simulink model "My_Nonlinear_Quaternions"  (R2021b)
settings: Solver=VariableStepAuto  StartTime=0.0  StopTime=simTime  RelTol=1e-3
undefined symbols (not defined in the file): b, D, g, k, L, m, MoI, omega, p, p_dot, quat, RPM, TakeStep
settings Model: Creator=Wojciech  LastModifiedBy=tanzc

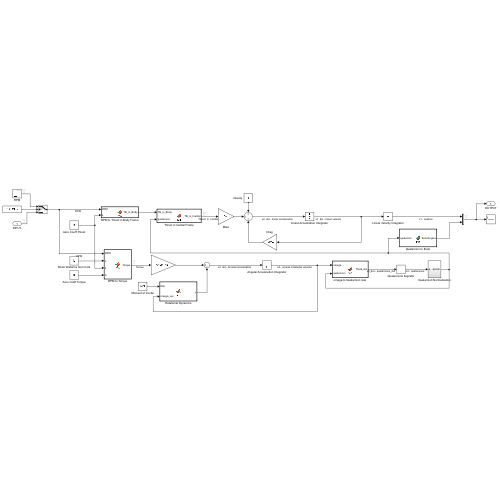
[thumbnail: Simulink's stored preview of the top-level diagram]
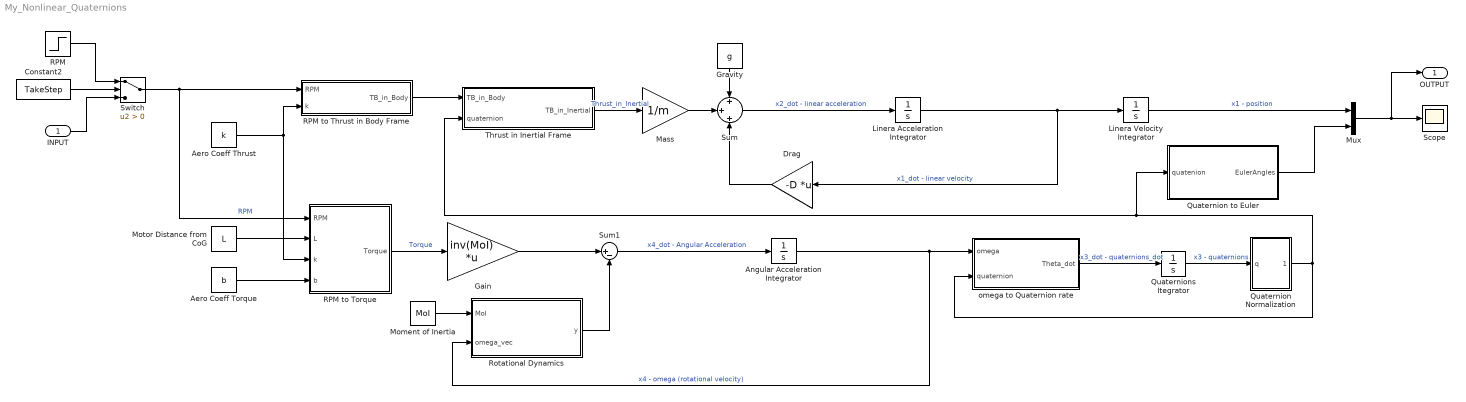
== system My_Nonlinear_Quaternions ==
  INPUT : Inport  PortDimensions=4
  Aero Coeff Thrust : Constant  Value=k
  Aero Coeff Torque : Constant  Value=b
  Angular Acceleration Integrator : Integrator  Priority=4  InitialCondition=omega
  Constant2 : Constant  Value=TakeStep
  Drag : Gain  Gain=-D  Multiplication=Matrix(K*u)
  Gain : Gain  Gain=inv(MoI)  Multiplication=Matrix(K*u)
  Gravity : Constant  Value=g  VectorParams1D=off
  Linera Acceleration Integrator : Integrator  Priority=2  InitialCondition=p_dot
  Linera Velocity Integrator : Integrator  Priority=1  InitialCondition=p
  Mass : Gain  Gain=1/m
  Moment of Inertia : Constant  Value=MoI  VectorParams1D=off
  Motor Distance from CoG : Constant  Value=L
  Mux : Mux  Inputs=2
  Quaternion Normalization : Subsystem
  Quaternion to Euler : MATLAB Function  TreatAsAtomicUnit=on
  Quaternions Itegrator : Integrator  Priority=3  InitialCondition=quat
  RPM : Step  Time=0  After=RPM  SampleTime=0
  RPM to Thrust in Body Frame : MATLAB Function  TreatAsAtomicUnit=on
  RPM to Torque : MATLAB Function  TreatAsAtomicUnit=on
  Rotational Dynamics : MATLAB Function  TreatAsAtomicUnit=on
  Scope : Scope
  Sum : Sum  Inputs=+|+|+
  Sum1 : Sum  Inputs=|+-
  Switch : Switch  Criteria=u2 > Threshold
  Thrust in Inertial Frame : MATLAB Function  TreatAsAtomicUnit=on
  "omega to Quaternion rate " : MATLAB Function  TreatAsAtomicUnit=on
  OUTPUT : Outport
  wires:
  Linera Velocity Integrator/1 -> Mux/1  "x1 - position"
  Linera Acceleration Integrator/1 -> Drag/1, Linera Velocity Integrator/1  "x1_dot - linear velocity"
  Sum/1 -> Linera Acceleration Integrator/1  "x2_dot - linear acceleration"
  Gravity/1 -> Sum/1
  RPM to Thrust in Body Frame/1(TB_in_Body) -> Thrust in Inertial Frame/1(TB_in_Body)
  Aero Coeff Thrust/1 -> RPM to Thrust in Body Frame/2(k), RPM to Torque/3(k)
  Thrust in Inertial Frame/1(TB_in_Inertial) -> Mass/1  "Thrust_in_Inertial"
  Mass/1 -> Sum/2
  Drag/1 -> Sum/3
  Motor Distance from CoG/1 -> RPM to Torque/2(L)
  Aero Coeff Torque/1 -> RPM to Torque/4(b)
  RPM to Torque/1(Torque) -> Gain/1  "Torque"
  Gain/1 -> Sum1/1
  Rotational Dynamics/1(y) -> Sum1/2
  Moment of Inertia/1 -> Rotational Dynamics/1(MoI)
  Sum1/1 -> Angular Acceleration Integrator/1  "x4_dot - Angular Acceleration"
  Angular Acceleration Integrator/1 -> "omega to Quaternion rate "/1(omega), Rotational Dynamics/2(omega_vec)  "x4 - omega (rotational velocity)"
  "omega to Quaternion rate "/1(Theta_dot) -> Quaternions Itegrator/1  "x3_dot - quaternions_dot"
  Quaternions Itegrator/1 -> Quaternion Normalization/1(q)  "x3 - quaternions"
  Mux/1 -> OUTPUT/1, Scope/1
  Constant2/1 -> Switch/2
  INPUT/1 -> Switch/3
  RPM/1 -> Switch/1
  Switch/1 -> RPM to Thrust in Body Frame/1(RPM), RPM to Torque/1(RPM)  "RPM"
  Quaternion Normalization/1(qnorm) -> Quaternion to Euler/1(quatenion), Thrust in Inertial Frame/2(quaternion), "omega to Quaternion rate "/2(quaternion)
  Quaternion to Euler/1(EulerAngles) -> Mux/2

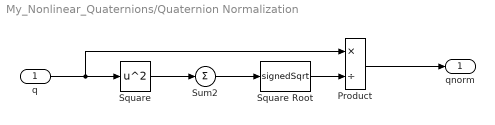
== system My_Nonlinear_Quaternions/Quaternion Normalization ==
  q : Inport  PortDimensions=4
  Product : Product  Inputs=*/
  Square : Math  Operator=square  SaturateOnIntegerOverflow=on
  Square Root : Sqrt  Operator=signedSqrt  SaturateOnIntegerOverflow=on
  Sum2 : Sum  Inputs=1
  qnorm : Outport  PortDimensions=4
  wires:
  Square Root/1 -> Product/2
  q/1 -> Product/1, Square/1
  Square/1 -> Sum2/1
  Sum2/1 -> Square Root/1
  Product/1 -> qnorm/1

== matlab function My_Nonlinear_Quaternions/RPM to Thrust in Body Frame ==
  data: RPM input; TB_in_Body output; k input
function TB_in_Body = fcn(RPM, k)
TB_in_Body = k * [0; 0; RPM'*RPM];

== matlab function My_Nonlinear_Quaternions/Thrust in Inertial Frame ==
  data: TB_in_Body input; quaternion input; TB_in_Inertial output
function TB_in_Inertial = fcn(TB_in_Body, quaternion)

% quaternion = [q0, q1, q2, q3]

q0 = quaternion(1);
q1 = quaternion(2);
q2 = quaternion(3);
q3 = quaternion(4);

R = quat2rotm([q0, q1, q2, q3]);

TB_in_Inertial = R*TB_in_Body;

== matlab function My_Nonlinear_Quaternions/RPM to Torque ==
  data: RPM input; Torque output; L input; k input; b input
function Torque = fcn(RPM, L, k, b)

Torque = [  L*k*(RPM(1)^2 - RPM(3)^2); ...
            L*k*(RPM(2)^2 - RPM(4)^2); ...
            b * (RPM(1)^2 - RPM(2)^2 + RPM(3)^2 - RPM(4)^2)];

== matlab function My_Nonlinear_Quaternions/Rotational Dynamics ==
  data: MoI input; omega_vec input; y output
function y = fcn(MoI, omega_vec)
Ixx = MoI(1,1);
Iyy = MoI(2,2);
Izz = MoI(3,3);

omega_x = omega_vec(1);
omega_y = omega_vec(2);
omega_z = omega_vec(3);

y = [ (Iyy-Izz)/Ixx*omega_y*omega_z; ...
      (Izz-Ixx)/Iyy*omega_x*omega_z; ...
      (Ixx-Iyy)/Izz*omega_x*omega_y];

== matlab function My_Nonlinear_Quaternions/omega to Quaternion rate  ==
  data: omega input; Theta_dot output; quaternion input
function Theta_dot = fcn(omega, quaternion)

q0 = quaternion(1);
q1 = quaternion(2);
q2 = quaternion(3);
q3 = quaternion(4);

w = [0; omega];

T = [ q0, -q1, -q2, -q3;
      q1, q0, -q3, q2;
      q2, q3, q0, -q1;
      q3, -q2, q1, q0];
  
Theta_dot = 0.5 * T * w;

== matlab function My_Nonlinear_Quaternions/Quaternion to Euler ==
  data: quatenion input; EulerAngles output
function EulerAngles = fcn(quatenion)

q0 = quatenion(1);
q1 = quatenion(2);
q2 = quatenion(3);
q3 = quatenion(4);

R = quat2rotm([q0, q1, q2, q3]);

psi = atan2(R(2,1), R(1,1));
theta = asin(-R(3, 1));
phi = atan2(R(3,2), R(3,3));

EulerAngles = [phi, theta, psi]';
